simulink model "hand_dryer_controller"  (R2024b)
settings: Solver=FixedStepDiscrete  StartTime=0.0  StopTime=inf  FixedStep=0.1  RelTol=1e-3
PostLoadFcn:
  | run("DesiredSolverSetting.m")
settings Model: Creator=ACER  LastModifiedBy=ACER

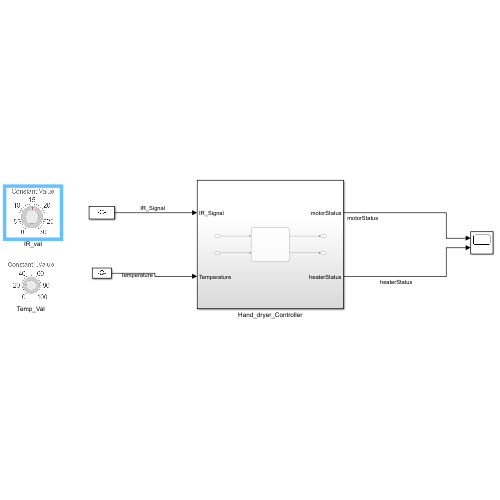
[thumbnail: Simulink's stored preview of the top-level diagram]
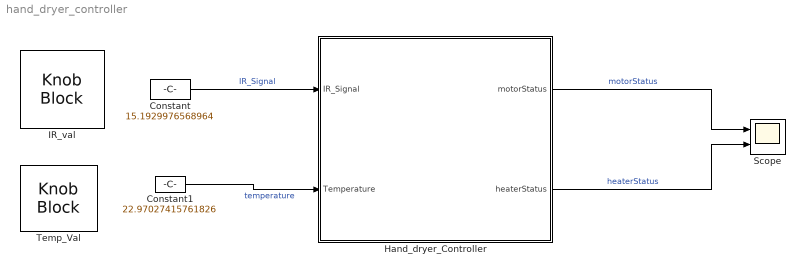
== system hand_dryer_controller ==
  Constant : Constant  Value=15.1929976568964
  Constant1 : Constant  Value=22.97027415761826
  Hand_dryer_Controller : Subsystem
  IR_val : KnobBlock  ScaleMax=30  TickInterval=5
  Scope : Scope  NumInputPorts=2
  Temp_Val : KnobBlock
  wires:
  Constant/1 -> Hand_dryer_Controller/1(IR_Signal)  "IR_Signal"
  Constant1/1 -> Hand_dryer_Controller/2(Temperature)  "temperature"
  Hand_dryer_Controller/1(motorStatus) -> Scope/1  "motorStatus"
  Hand_dryer_Controller/2(heaterStatus) -> Scope/2  "heaterStatus"

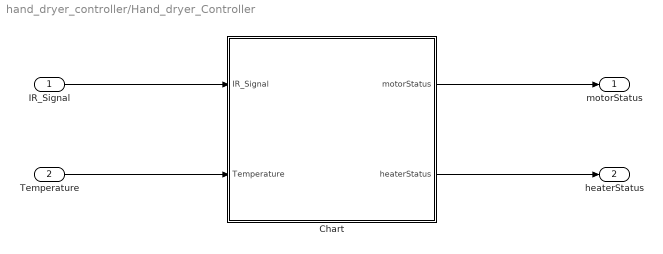
== system hand_dryer_controller/Hand_dryer_Controller ==
  IR_Signal : Inport
  Temperature : Inport  Port=2
  Chart : Stateflow chart  TreatAsAtomicUnit=on
  motorStatus : Outport  OutDataTypeStr=Enum: Status
  heaterStatus : Outport  Port=2  OutDataTypeStr=Enum: Status
  wires:
  IR_Signal/1 -> Chart/1(IR_Signal)
  Temperature/1 -> Chart/2(Temperature)
  Chart/1(motorStatus) -> motorStatus/1
  Chart/2(heaterStatus) -> heaterStatus/1

== stateflow chart hand_dryer_controller/Hand_dryer_Controller/Chart ==
  state highTemp
    en:
    motorStatus = On;
    heaterStatus = Off;
  note: /* For this model we are going to use step time of 0.1 s. So for debounce time of 0.5 second counter will count till 5 */
  state Idle
    en:
    motorStatus = Off;
    heaterStatus = Off;
  state debounce_logic
    en:
    count = 0;
    du:
    count=count+1;
  state Active
    en:
    motorStatus=On;
    heaterStatus = On;
  state debounce_logic_2
    en:
    count=0;
    du:
    count = count+1;
  (default) -> Idle
  Active -> highTemp [order 2] : [Temperature>=70]
  highTemp -> Active [order 2] : [Temperature<65]
  highTemp -> debounce_logic_2 [order 1] : [IR_Signal>10]
  Idle -> debounce_logic : [IR_Signal<=10]
  Active -> debounce_logic_2 [order 1] : [IR_Signal>10]
  debounce_logic -> Active [order 2] : [count>5]
  debounce_logic_2 -> Active [order 1] : [IR_Signal<10]
  debounce_logic -> Idle [order 1] : [IR_Signal>10]
  debounce_logic_2 -> Idle [order 2] : [count>5]
  data: IR_Signal input; Temperature input; motorStatus output Enum: Status; heaterStatus output Enum: Status; count local
